simulink model "Longitudinal_Control"  (R2024a)
settings: Solver=VariableStepAuto  StartTime=0.0  StopTime=30  RelTol=1e-3
libraries: simulink x1
settings Model: Creator=28126  LastModifiedBy=28126

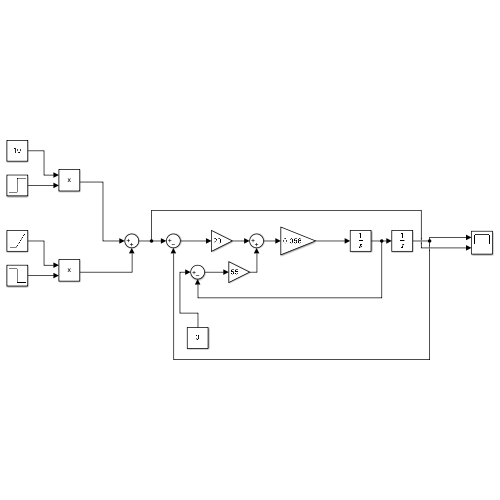
[thumbnail: Simulink's stored preview of the top-level diagram]
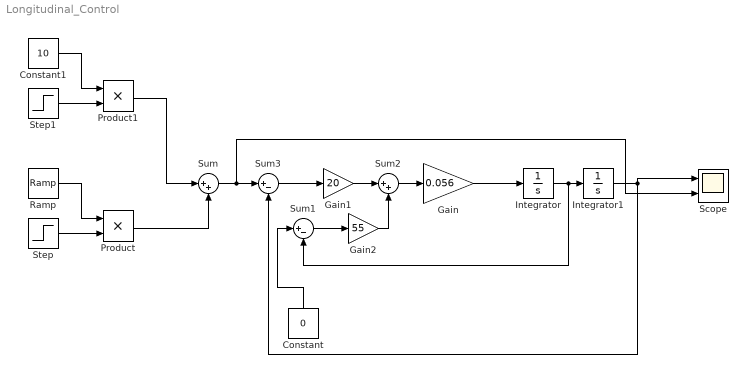
== system Longitudinal_Control ==
  Constant : Constant  Value=0
  Constant1 : Constant  Value=10
  Gain : Gain  Gain=0.056
  Gain1 : Gain  Gain=20
  Gain2 : Gain  Gain=55
  Integrator : Integrator
  Integrator1 : Integrator
  Product : Product
  Product1 : Product
  Ramp : simulink/Sources/Ramp  slope=1  start=0  InitialOutput=0
  Scope : Scope  NumInputPorts=2
  Step : Step  Time=10  Before=1  After=0  SampleTime=0
  Step1 : Step  Time=10  SampleTime=0
  Sum : Sum  Inputs=|++
  Sum1 : Sum  Inputs=|+-
  Sum2 : Sum  Inputs=|++
  Sum3 : Sum  Inputs=|+-
  wires:
  Gain/1 -> Integrator/1
  Integrator/1 -> Sum1/2, Integrator1/1
  Integrator1/1 -> Sum3/2, Scope/1
  Sum1/1 -> Gain2/1
  Gain1/1 -> Sum2/1
  Sum2/1 -> Gain/1
  Gain2/1 -> Sum2/2
  Constant/1 -> Sum1/1
  Step/1 -> Product/2
  Ramp/1 -> Product/1
  Step1/1 -> Product1/2
  Constant1/1 -> Product1/1
  Product1/1 -> Sum/1
  Product/1 -> Sum/2
  Sum3/1 -> Gain1/1
  Sum/1 -> Scope/2, Sum3/1
